simulink model "sampleModel106"  (R2022a)
settings: Solver=VariableStepAuto  StartTime=0.0  StopTime=10.0  RelTol=1e-3
undefined symbols (not defined in the file): DiscIntNeverNeededParam, magnitude, Newton, Raphson
libraries: simulink x379, slpidlib x89
(part 11 of 16)

== system sampleModel106/cfblk80/cfblk10/cfblk8/cfblk12 ==
  cfblk1 : Inport
  cfblk14 : Inport  Port=2
  Action Port : ActionPort  ActionPortLabel=if(u1 >= 0)
  cfblk10 : ComplexToRealImag
  cfblk11 : Constant  Value=[647263997.396458]  SampleTime=1
  cfblk12 : Constant  Value=[-710280411.344243]  SampleTime=1
  cfblk13 : Constant  Value=[-145557332.228966]  SampleTime=1
  cfblk18 : Delay
  cfblk19 : Delay
  cfblk20 : Delay
  cfblk3 : slpidlib/PID Controller (2DOF)  Controller=PID  Form=Parallel  TimeDomain=Discrete-time  UseExternalTs=off  SampleTime=-1  IntegratorMethod=Forward Euler  FilterMethod=Forward Euler  ControllerParametersSource=internal  P=1  I=1  UseKiTs=off  D=0  N=100  UseFilter=on  b=1  c=1  TunerSelectOption=Transfer Function Based (PID Tuner App)  InitialConditionSource=internal  InitialConditionForIntegrator=0  InitialConditionForFilter=0  DifferentiatorICPrevScaledInput=0  ExternalReset=none  TrackingMode=off  Kt=1  LimitOutput=off  SatLimitsSource=internal  UpperSaturationLimit=inf  LowerSaturationLimit=-inf  LinearizeAsGain=off  AntiWindupMode=none  Kb=1  POutMin=[]  POutMax=[]  IOutMin=[]  IOutMax=[]  DOutMin=[]  DOutMax=[]  NOutMin=[]  NOutMax=[]  bOutMin=[]  bOutMax=[]  cOutMin=[]  cOutMax=[]  SumOutMin=[]  SumOutMax=[]  SaturationOutMin=[]  SaturationOutMax=[]  PParamMin=[]  PParamMax=[]  IParamMin=[]  IParamMax=[]  DParamMin=[]  DParamMax=[]  NParamMin=[]  NParamMax=[]  bParamMin=[]  bParamMax=[]  cParamMin=[]  cParamMax=[]  KbParamMin=[]  KbParamMax=[]  KtParamMin=[]  KtParamMax=[]  KbOutMin=[]  KbOutMax=[]  KtOutMin=[]  KtOutMax=[]  IntegratorOutMin=[]  IntegratorOutMax=[]  FilterOutMin=[]  FilterOutMax=[]  SumI1OutMin=[]  SumI1OutMax=[]  SumI2OutMin=[]  SumI2OutMax=[]  SumI3OutMin=[]  SumI3OutMax=[]  SumI4OutMin=[]  SumI4OutMax=[]  SumDOutMin=[]  SumDOutMax=[]  Sum1OutMin=[]  Sum1OutMax=[]  Sum2OutMin=[]  Sum2OutMax=[]  Sum3OutMin=[]  Sum3OutMax=[]  DifferentiatorOutMin=[]  DifferentiatorOutMax=[]  FilterDiffOutCoefMin=[]  FilterDiffOutCoefMax=[]  ReciprocalOutMin=[]  ReciprocalOutMax=[]  SumDenOutMin=[]  SumDenOutMax=[]  SumNumOutMin=[]  SumNumOutMax=[]  DivideOutMin=[]  DivideOutMax=[]  UdiffTsProdOutMin=[]  UdiffTsProdOutMax=[]  NTsProdOutMin=[]  NTsProdOutMax=[]  UintegralTsProdOutMin=[]  UintegralTsProdOutMax=[]  UngainTsProdOutMin=[]  UngainTsProdOutMax=[]  IntegratorContinuousStateAttributes=''  IntegratorStateMustResolveToSignalObject=off  IntegratorRTWStateStorageClass=Auto  FilterContinuousStateAttributes=''  FilterStateMustResolveToSignalObject=off  FilterRTWStateStorageClass=Auto  ParallelPVariant=InternalParameters  IdealPVariant=Disabled  IVariant=InternalParameters  DVariant=InternalParameters  bVariant=InternalParameters  cVariant=InternalParameters  IntegratorVariant=Discrete  SatVariant=Disabled  AWVariant=Passthrough  PCopyVariant=Disabled  TRVariant=Disabled  FdbkBlocksVariant=Forward  IdealPFdbkVariant=Disabled  SatFdbkVariant=Disabled  DerivativeFilterVariant=ForwardEulerFilter  NVariant=InternalParameters  NCopyVariant=Disabled  FilterICVariant=InternalICsFilter  IntegratorICVariant=InternalICs  ExternalResetVariant=Disabled  TRSumVariant=Passthrough  SumFdbkVariant=Disabled  SumVariant=Sum_PID  TsampFilterVariant=InternalTs  TsampNgainVariant=Passthrough  TsampIntegralVariant=Passthrough  ExternalSaturationOutDataTypeStr=Inherit: Same as second input
      settings: SourceProductBaseCode=SL
  cfblk4 : Squeeze
  cfblk5 : Sum  Inputs=+-
  cfblk6 : Sum  Inputs=+-
  cfblk7 : Sum  Inputs=|++
  cfblk8 : Sum  Inputs=+
  cfblk9 : ComplexToRealImag
  cfblk2 : Outport
  cfblk15 : Outport  Port=2
  cfblk16 : Outport  Port=3
  cfblk17 : Outport  Port=4
  wires:
  cfblk9/1 -> cfblk15/1
  cfblk13/1 -> cfblk17/1
  cfblk3/1 -> cfblk5/1
  cfblk14/1 -> cfblk2/1
  cfblk5/1 -> cfblk7/1
  cfblk9/2 -> cfblk10/1, cfblk6/2
  cfblk7/1 -> cfblk8/1
  cfblk8/1 -> cfblk9/1
  cfblk4/1 -> cfblk16/1
  cfblk12/1 -> cfblk7/2
  cfblk11/1 -> cfblk6/1
  cfblk1/1 -> cfblk4/1
  cfblk10/1 -> cfblk18/1
  cfblk18/1 -> cfblk3/1
  cfblk10/2 -> cfblk19/1
  cfblk19/1 -> cfblk3/2
  cfblk6/1 -> cfblk20/1
  cfblk20/1 -> cfblk5/2

== system sampleModel106/cfblk80/cfblk10/cfblk8/cfblk13 ==
  cfblk1 : Inport
  cfblk13 : Inport  Port=2
  cfblk14 : Inport  Port=3
  cfblk15 : Inport  Port=4
  cfblk16 : Inport  Port=5
  cfblk17 : Inport  Port=6
  Action Port : ActionPort  ActionPortLabel=else
  cfblk10 : Constant  Value=[-897843886.378087]  SampleTime=1
  cfblk11 : Constant  Value=[302517880.201654]  SampleTime=1
  cfblk12 : Constant  Value=[630403089.803577]  SampleTime=1
  cfblk3 : simulink/Discrete/Transfer Fcn Real Zero  ZeroZ=0.75  ICPrevInput=0.0  DoSatur=off
      settings: SourceProductBaseCode=SL
  cfblk4 : Reshape
  cfblk5 : Signum
  cfblk6 : Squeeze
  cfblk7 : Bias  Bias=[473175821.464954]  SaturateOnIntegerOverflow=off
  cfblk8 : PermuteDimensions
  cfblk9 : Constant  Value=[-532839668.441266]  SampleTime=1
  cfblk2 : Outport
  wires:
  cfblk11/1 -> cfblk5/1
  cfblk3/1 -> cfblk8/1
  cfblk1/1 -> cfblk3/1
  cfblk9/1 -> cfblk6/1
  cfblk16/1 -> cfblk4/1
  cfblk17/1 -> cfblk2/1
  cfblk15/1 -> cfblk7/1

== system sampleModel106/cfblk80/cfblk10/cfblk8/cfblk6 ==
  cfblk1 : Inport
  cfblk8 : Inport  Port=2
  cfblk9 : Inport  Port=3
  cfblk10 : Inport  Port=4
  cfblk3 : simulink/Discrete/Difference  ICPrevInput=0.0  OutMin=[]  OutMax=[]  OutDataTypeStr=Inherit: Inherit via back propagation  OutDataType=fixdt(1, 16)  OutScaling=2^-10  DoSatur=off
  cfblk4 : Trigonometry
  cfblk5 : Sum  Inputs=+-
  cfblk6 : Constant  Value=[-342792369.326935]  SampleTime=1
  cfblk7 : Constant  Value=[-642019709.076268]  SampleTime=1
  cfblk2 : Outport
  wires:
  cfblk3/1 -> cfblk2/1
  cfblk7/1 -> cfblk5/1
  cfblk10/1 -> cfblk5/2
  cfblk6/1 -> cfblk4/1
  cfblk4/1 -> cfblk3/1

== system sampleModel106/cfblk80/cfblk10/cfblk8/cfblk7 ==
  cfblk1 : Inport
  cfblk15 : Inport  Port=2
  cfblk16 : Inport  Port=3
  cfblk10 : Sum  Inputs=+-
  cfblk11 : Constant  Value=[-15116580.989043]  SampleTime=1
  cfblk12 : Constant  Value=[685298469.116732]  SampleTime=1
  cfblk13 : Constant  Value=[-327896226.329159]  SampleTime=1
  cfblk14 : Constant  Value=[801147045.676296]  SampleTime=1
  cfblk17 : Delay  SampleTime=1
  cfblk3 : Bias  Bias=[-977258308.912659]  SaturateOnIntegerOverflow=off
  cfblk4 : Sum  Inputs=+-
  cfblk5 : Polyval  Coefs=[ +2.081618890e-019, -1.441693666e-014, +4.719686976e-010, -8.536869453e-006, +1.621573104e-001, -8.087801117e+001 ]
  cfblk6 : simulink/Math Operations/MinMax Running Resettable  Function=min  vinit=0.0
  cfblk7 : MinMax  Inputs=2
  cfblk8 : simulink/Math Operations/MinMax Running Resettable  Function=min  vinit=0.0
  cfblk9 : Sin  TimeSource=Use external signal  SampleTime=0
  cfblk2 : Outport
  wires:
  cfblk4/1 -> cfblk7/1
  cfblk13/1 -> cfblk7/2
  cfblk12/1 -> cfblk2/1
  cfblk5/1 -> cfblk4/1
  cfblk3/1 -> cfblk5/1
  cfblk10/1 -> cfblk6/1
  cfblk9/1 -> cfblk6/2
  cfblk14/1 -> cfblk8/1
  cfblk15/1 -> cfblk8/2
  cfblk1/1 -> cfblk3/1
  cfblk8/1 -> cfblk9/1
  cfblk16/1 -> cfblk4/2
  cfblk7/1 -> cfblk10/1
  cfblk6/1 -> cfblk17/1
  cfblk17/1 -> cfblk10/2

== system sampleModel106/cfblk80/cfblk10/cfblk8/cfblk8 ==
  cfblk1 : Inport
  cfblk7 : Inport  Port=2
  cfblk8 : Inport  Port=3
  cfblk9 : Inport  Port=4
  cfblk3 : UnitDelay  HasFrameUpgradeWarning=on
  cfblk4 : Signum
  cfblk5 : Sqrt  Operator=rSqrt  AlgorithmType=Newton-Raphson
  cfblk6 : simulink/Math Operations/MinMax Running Resettable  Function=min  vinit=0.0
  cfblk2 : Outport
  cfblk10 : Outport  Port=2
  cfblk11 : Outport  Port=3
  cfblk12 : Outport  Port=4
  wires:
  cfblk7/1 -> cfblk5/1
  cfblk8/1 -> cfblk3/1
  cfblk3/1 -> cfblk4/1, cfblk2/1
  cfblk6/1 -> cfblk10/1
  cfblk1/1 -> cfblk11/1
  cfblk4/1 -> cfblk12/1
  cfblk5/1 -> cfblk6/1
  cfblk9/1 -> cfblk6/2

== system sampleModel106/cfblk80/cfblk10/cfblk8/cfblk9 ==
  cfblk1 : Inport
  cfblk7 : Inport  Port=2
  cfblk10 : Delay  SampleTime=1
  cfblk11 : Delay  SampleTime=1
  cfblk3 : DiscreteZeroPole  Poles=[0 0.5]  Gain=1
  cfblk4 : UnaryMinus
  cfblk5 : simulink/Math Operations/MinMax Running Resettable  Function=min  vinit=0.0
  cfblk6 : Product  Inputs=**
  cfblk2 : Outport
  cfblk8 : Outport  Port=2
  cfblk9 : Outport  Port=3
  wires:
  cfblk4/1 -> cfblk6/1
  cfblk5/1 -> cfblk2/1, cfblk4/1
  cfblk7/1 -> cfblk8/1
  cfblk6/1 -> cfblk3/1, cfblk11/1
  cfblk1/1 -> cfblk5/1, cfblk9/1
  cfblk3/1 -> cfblk10/1
  cfblk10/1 -> cfblk6/2
  cfblk11/1 -> cfblk5/2

== system sampleModel106/cfblk80/cfblk10/cfblk9/cfblk8 ==
  cfblk1 : Inport
  cfblk7 : Inport  Port=2
  cfblk8 : Inport  Port=3
  cfblk9 : Inport  Port=4
  cfblk3 : simulink/Discrete/Transfer Fcn First Order  PoleZ=0.95  ICPrevOutput=0.0  DoSatur=off
  cfblk4 : Abs  SaturateOnIntegerOverflow=off
  cfblk5 : Sum  Inputs=+
  cfblk6 : Constant  Value=[-161739607.877266]  SampleTime=1
  cfblk2 : Outport
  cfblk10 : Outport  Port=2
  wires:
  cfblk8/1 -> cfblk2/1
  cfblk3/1 -> cfblk5/1
  cfblk4/1 -> cfblk10/1
  cfblk7/1 -> cfblk3/1
  cfblk5/1 -> cfblk4/1

== system sampleModel106/cfblk80/cfblk10/cfblk9/cfblk9 ==
  cfblk1 : Inport
  cfblk3 : simulink/Discrete/Transfer Fcn Lead or Lag  PoleZ=0.95  ZeroZ=0.75  ICPrevOutput=0.0  ICPrevInput=0.0  DoSatur=off
      settings: SourceProductBaseCode=SL
  cfblk4 : Product  Inputs=*
  cfblk5 : Sum
  cfblk6 : Bias  Bias=[-67652395.251411]  SaturateOnIntegerOverflow=off
  cfblk2 : Outport
  cfblk7 : Outport  Port=2
  wires:
  cfblk6/1 -> cfblk5/1
  cfblk1/1 -> cfblk2/1, cfblk3/1, cfblk6/1
  cfblk3/1 -> cfblk4/1
  cfblk5/1 -> cfblk7/1
  cfblk4/1 -> cfblk5/2

== system sampleModel106/cfblk80/cfblk11/cfblk10/cfblk8 ==
  cfblk1 : Inport
  cfblk8 : Inport  Port=2
  cfblk3 : Product  Inputs=**
  cfblk4 : ComplexToRealImag
  cfblk5 : Sqrt  Operator=rSqrt  AlgorithmType=Newton-Raphson
  cfblk6 : ComplexToRealImag
  cfblk7 : Constant  Value=[634238120.262405]  SampleTime=1
  cfblk2 : Outport
  cfblk9 : Outport  Port=2
  wires:
  cfblk7/1 -> cfblk5/1
  cfblk6/1 -> cfblk9/1
  cfblk4/1 -> cfblk3/1
  cfblk1/1 -> cfblk6/1
  cfblk8/1 -> cfblk4/1
  cfblk6/2 -> cfblk2/1
  cfblk5/1 -> cfblk3/2

== system sampleModel106/cfblk80/cfblk11/cfblk10/cfblk9 ==
  cfblk1 : Inport
  cfblk6 : Inport  Port=2
  cfblk3 : Product  Inputs=**
  cfblk4 : Sqrt
  cfblk5 : Constant  Value=[-951789806.354500]  SampleTime=1
  cfblk2 : Outport
  cfblk7 : Outport  Port=2
  wires:
  cfblk4/1 -> cfblk7/1
  cfblk5/1 -> cfblk3/1
  cfblk3/1 -> cfblk4/1
  cfblk6/1 -> cfblk3/2
  cfblk1/1 -> cfblk2/1

== system sampleModel106/cfblk80/cfblk11/cfblk8/cfblk10 ==
  cfblk1 : Inport
  cfblk10 : Inport  Port=2
  cfblk11 : Inport  Port=3
  cfblk13 : Delay  SampleTime=1
  cfblk3 : DiscreteZeroPole  Poles=[0 0.5]  Gain=1
  cfblk4 : Product  Inputs=**
  cfblk5 : Sum  Inputs=+
  cfblk6 : Sqrt
  cfblk7 : simulink/Math Operations/Slider Gain  gain=1  low=0  high=2
  cfblk8 : Gain  Gain=[838906056.735311]
  cfblk9 : Constant  Value=[952501991.848955]  SampleTime=1
  cfblk2 : Outport
  cfblk12 : Outport  Port=2
  wires:
  cfblk9/1 -> cfblk4/1
  cfblk5/1 -> cfblk6/1
  cfblk7/1 -> cfblk3/1
  cfblk8/1 -> cfblk12/1
  cfblk3/1 -> cfblk2/1
  cfblk11/1 -> cfblk7/1
  cfblk4/1 -> cfblk5/1
  cfblk10/1 -> cfblk8/1
  cfblk6/1 -> cfblk13/1
  cfblk13/1 -> cfblk4/2

== system sampleModel106/cfblk80/cfblk11/cfblk8/cfblk11 ==
  cfblk1 : Inport
  cfblk10 : Constant  Value=[-97826944.029732]  SampleTime=1
  cfblk3 : simulink/Math Operations/Slider Gain  gain=1  low=0  high=2
  cfblk4 : Sum  Inputs=|++
  cfblk5 : Sum  Inputs=+-
  cfblk6 : Trigonometry
  cfblk7 : Reshape
  cfblk8 : Constant  Value=[564328220.436240]  SampleTime=1
  cfblk9 : Constant  Value=[-958432842.586397]  SampleTime=1
  cfblk2 : Outport
  cfblk11 : Outport  Port=2
  cfblk12 : Outport  Port=3
  wires:
  cfblk8/1 -> cfblk4/1
  cfblk4/1 -> cfblk7/1
  cfblk10/1 -> cfblk12/1, cfblk3/1
  cfblk6/1 -> cfblk5/1
  cfblk3/1 -> cfblk6/1
  cfblk9/1 -> cfblk5/2
  cfblk1/1 -> cfblk2/1
  cfblk5/1 -> cfblk4/2
  cfblk7/1 -> cfblk11/1

== system sampleModel106/cfblk80/cfblk11/cfblk8/cfblk12 ==
  cfblk1 : Inport
  cfblk10 : Inport  Port=2
  cfblk11 : Inport  Port=3
  cfblk12 : Inport  Port=4
  cfblk14 : Delay  SampleTime=1
  cfblk3 : slpidlib/PID Controller  Controller=PID  Form=Parallel  TimeDomain=Discrete-time  UseExternalTs=off  SampleTime=1  IntegratorMethod=Forward Euler  FilterMethod=Forward Euler  ControllerParametersSource=internal  P=1  I=1  UseKiTs=off  D=0  N=100  UseFilter=on  TunerSelectOption=Transfer Function Based (PID Tuner App)  InitialConditionSource=internal  InitialConditionForIntegrator=0  InitialConditionForFilter=0  DifferentiatorICPrevScaledInput=0  ExternalReset=none  TrackingMode=off  Kt=1  LimitOutput=off  SatLimitsSource=internal  UpperSaturationLimit=inf  LowerSaturationLimit=-inf  LinearizeAsGain=off  AntiWindupMode=none  Kb=1  POutMin=[]  POutMax=[]  IOutMin=[]  IOutMax=[]  DOutMin=[]  DOutMax=[]  NOutMin=[]  NOutMax=[]  SumOutMin=[]  SumOutMax=[]  SaturationOutMin=[]  SaturationOutMax=[]  PParamMin=[]  PParamMax=[]  IParamMin=[]  IParamMax=[]  DParamMin=[]  DParamMax=[]  NParamMin=[]  NParamMax=[]  KbParamMin=[]  KbParamMax=[]  KtParamMin=[]  KtParamMax=[]  KbOutMin=[]  KbOutMax=[]  KtOutMin=[]  KtOutMax=[]  IntegratorOutMin=[]  IntegratorOutMax=[]  FilterOutMin=[]  FilterOutMax=[]  SumI1OutMin=[]  SumI1OutMax=[]  SumI2OutMin=[]  SumI2OutMax=[]  SumI3OutMin=[]  SumI3OutMax=[]  SumI4OutMin=[]  SumI4OutMax=[]  SumDOutMin=[]  SumDOutMax=[]  DifferentiatorOutMin=[]  DifferentiatorOutMax=[]  FilterDiffOutCoefMin=[]  FilterDiffOutCoefMax=[]  ReciprocalOutMin=[]  ReciprocalOutMax=[]  SumDenOutMin=[]  SumDenOutMax=[]  SumNumOutMin=[]  SumNumOutMax=[]  DivideOutMin=[]  DivideOutMax=[]  UdiffTsProdOutMin=[]  UdiffTsProdOutMax=[]  NTsProdOutMin=[]  NTsProdOutMax=[]  UintegralTsProdOutMin=[]  UintegralTsProdOutMax=[]  UngainTsProdOutMin=[]  UngainTsProdOutMax=[]  IntegratorContinuousStateAttributes=''  IntegratorStateMustResolveToSignalObject=off  IntegratorRTWStateStorageClass=Auto  FilterContinuousStateAttributes=''  FilterStateMustResolveToSignalObject=off  FilterRTWStateStorageClass=Auto  ParallelPVariant=InternalParameters  IdealPVariant=Disabled  IVariant=InternalParameters  DVariant=InternalParameters  IntegratorVariant=Discrete  SatVariant=Disabled  AWVariant=Passthrough  PCopyVariant=Disabled  TRVariant=Disabled  FdbkBlocksVariant=Forward  IdealPFdbkVariant=Disabled  SatFdbkVariant=Disabled  DerivativeFilterVariant=ForwardEulerFilter  NVariant=InternalParameters  NCopyVariant=Disabled  FilterICVariant=InternalICsFilter  IntegratorICVariant=InternalICs  ExternalResetVariant=Disabled  TRSumVariant=Passthrough  SumFdbkVariant=Disabled  SumVariant=Sum_PID  TsampFilterVariant=InternalTs  TsampNgainVariant=Passthrough  TsampIntegralVariant=Passthrough  ExternalSaturationOutDataTypeStr=Inherit: Same as second input  aMode=0
  cfblk4 : Math  Operator=magnitude^2
  cfblk5 : Squeeze
  cfblk6 : Sum  Inputs=-+
  cfblk7 : simulink/Math Operations/Slider Gain  gain=1  low=0  high=2
  cfblk8 : PermuteDimensions
  cfblk9 : Constant  Value=[355141637.645424]  SampleTime=1
  cfblk2 : Outport
  cfblk13 : Outport  Port=2
  wires:
  cfblk11/1 -> cfblk4/1
  cfblk10/1 -> cfblk2/1
  cfblk12/1 -> cfblk8/1
  cfblk3/1 -> cfblk6/1
  cfblk1/1 -> cfblk13/1
  cfblk8/1 -> cfblk7/1
  cfblk4/1 -> cfblk6/2
  cfblk6/1 -> cfblk5/1
  cfblk5/1 -> cfblk14/1
  cfblk14/1 -> cfblk3/1

== system sampleModel106/cfblk80/cfblk11/cfblk8/cfblk7 ==
  cfblk1 : Inport
  cfblk7 : Inport  Port=2
  cfblk3 : simulink/Discrete/Difference  ICPrevInput=0.0  OutMin=[]  OutMax=[]  OutDataTypeStr=Inherit: Inherit via back propagation  OutDataType=fixdt(1, 16)  OutScaling=2^-10  DoSatur=off
  cfblk4 : Constant  Value=[-388420622.706026]  SampleTime=1
  cfblk5 : Constant  Value=[174605432.981955]  SampleTime=1
  cfblk6 : Constant  Value=[-811978133.934877]  SampleTime=1
  cfblk2 : Outport
  wires:
  cfblk1/1 -> cfblk2/1
  cfblk6/1 -> cfblk3/1

== system sampleModel106/cfblk80/cfblk11/cfblk8/cfblk8 ==
  cfblk1 : Inport
  cfblk13 : Inport  Port=2
  cfblk14 : Inport  Port=3
  cfblk15 : Inport  Port=4
  cfblk10 : Product
  cfblk11 : Signum
  cfblk12 : Polyval  Coefs=[ +2.081618890e-019, -1.441693666e-014, +4.719686976e-010, -8.536869453e-006, +1.621573104e-001, -8.087801117e+001 ]
  cfblk16 : Delay  SampleTime=1
  cfblk3 : simulink/Discrete/Tapped Delay  vinit=0.0  samptime=-1  NumDelays=1  DelayOrder=Oldest  includeCurrent=off
  cfblk4 : simulink/Discrete/Transfer Fcn Lead or Lag  PoleZ=0.95  ZeroZ=0.75  ICPrevOutput=0.0  ICPrevInput=0.0  DoSatur=off
      settings: SourceProductBaseCode=SL
  cfblk5 : slpidlib/PID Controller (2DOF)  Controller=PID  Form=Parallel  TimeDomain=Discrete-time  UseExternalTs=off  SampleTime=1  IntegratorMethod=Forward Euler  FilterMethod=Forward Euler  ControllerParametersSource=internal  P=1  I=1  UseKiTs=off  D=0  N=100  UseFilter=on  b=1  c=1  TunerSelectOption=Transfer Function Based (PID Tuner App)  InitialConditionSource=internal  InitialConditionForIntegrator=0  InitialConditionForFilter=0  DifferentiatorICPrevScaledInput=0  ExternalReset=none  TrackingMode=off  Kt=1  LimitOutput=off  SatLimitsSource=internal  UpperSaturationLimit=inf  LowerSaturationLimit=-inf  LinearizeAsGain=off  AntiWindupMode=none  Kb=1  POutMin=[]  POutMax=[]  IOutMin=[]  IOutMax=[]  DOutMin=[]  DOutMax=[]  NOutMin=[]  NOutMax=[]  bOutMin=[]  bOutMax=[]  cOutMin=[]  cOutMax=[]  SumOutMin=[]  SumOutMax=[]  SaturationOutMin=[]  SaturationOutMax=[]  PParamMin=[]  PParamMax=[]  IParamMin=[]  IParamMax=[]  DParamMin=[]  DParamMax=[]  NParamMin=[]  NParamMax=[]  bParamMin=[]  bParamMax=[]  cParamMin=[]  cParamMax=[]  KbParamMin=[]  KbParamMax=[]  KtParamMin=[]  KtParamMax=[]  KbOutMin=[]  KbOutMax=[]  KtOutMin=[]  KtOutMax=[]  IntegratorOutMin=[]  IntegratorOutMax=[]  FilterOutMin=[]  FilterOutMax=[]  SumI1OutMin=[]  SumI1OutMax=[]  SumI2OutMin=[]  SumI2OutMax=[]  SumI3OutMin=[]  SumI3OutMax=[]  SumI4OutMin=[]  SumI4OutMax=[]  SumDOutMin=[]  SumDOutMax=[]  Sum1OutMin=[]  Sum1OutMax=[]  Sum2OutMin=[]  Sum2OutMax=[]  Sum3OutMin=[]  Sum3OutMax=[]  DifferentiatorOutMin=[]  DifferentiatorOutMax=[]  FilterDiffOutCoefMin=[]  FilterDiffOutCoefMax=[]  ReciprocalOutMin=[]  ReciprocalOutMax=[]  SumDenOutMin=[]  SumDenOutMax=[]  SumNumOutMin=[]  SumNumOutMax=[]  DivideOutMin=[]  DivideOutMax=[]  UdiffTsProdOutMin=[]  UdiffTsProdOutMax=[]  NTsProdOutMin=[]  NTsProdOutMax=[]  UintegralTsProdOutMin=[]  UintegralTsProdOutMax=[]  UngainTsProdOutMin=[]  UngainTsProdOutMax=[]  IntegratorContinuousStateAttributes=''  IntegratorStateMustResolveToSignalObject=off  IntegratorRTWStateStorageClass=Auto  FilterContinuousStateAttributes=''  FilterStateMustResolveToSignalObject=off  FilterRTWStateStorageClass=Auto  ParallelPVariant=InternalParameters  IdealPVariant=Disabled  IVariant=InternalParameters  DVariant=InternalParameters  bVariant=InternalParameters  cVariant=InternalParameters  IntegratorVariant=Discrete  SatVariant=Disabled  AWVariant=Passthrough  PCopyVariant=Disabled  TRVariant=Disabled  FdbkBlocksVariant=Forward  IdealPFdbkVariant=Disabled  SatFdbkVariant=Disabled  DerivativeFilterVariant=ForwardEulerFilter  NVariant=InternalParameters  NCopyVariant=Disabled  FilterICVariant=InternalICsFilter  IntegratorICVariant=InternalICs  ExternalResetVariant=Disabled  TRSumVariant=Passthrough  SumFdbkVariant=Disabled  SumVariant=Sum_PID  TsampFilterVariant=InternalTs  TsampNgainVariant=Passthrough  TsampIntegralVariant=Passthrough  ExternalSaturationOutDataTypeStr=Inherit: Same as second input
      settings: SourceProductBaseCode=SL
  cfblk6 : Delay  DelayLengthSource=Input port  SampleTime=1
      settings: InputPortMap=u0,p1
  cfblk7 : simulink/Discrete/Transfer Fcn Real Zero  ZeroZ=0.75  ICPrevInput=0.0  DoSatur=off
      settings: SourceProductBaseCode=SL
  cfblk8 : ComplexToMagnitudeAngle
  cfblk9 : ComplexToMagnitudeAngle
  cfblk2 : Outport
  wires:
  cfblk5/1 -> cfblk12/1
  cfblk6/1 -> cfblk2/1
  cfblk12/1 -> cfblk9/1
  cfblk4/1 -> cfblk3/1
  cfblk8/1 -> cfblk10/2
  cfblk11/1 -> cfblk8/1
  cfblk13/1 -> cfblk4/1
  cfblk1/1 -> cfblk11/1
  cfblk7/1 -> cfblk5/1
  cfblk10/1 -> cfblk5/2
  cfblk15/1 -> cfblk7/1
  cfblk3/1 -> cfblk6/1
  cfblk8/2 -> cfblk6/2
  cfblk9/1 -> cfblk16/1
  cfblk16/1 -> cfblk10/1

== system sampleModel106/cfblk80/cfblk11/cfblk8/cfblk9 ==
  cfblk1 : Inport
  cfblk11 : Inport  Port=2
  cfblk12 : Inport  Port=3
  cfblk13 : Inport  Port=4
  cfblk14 : Inport  Port=5
  cfblk10 : Math  Operator=rem
  cfblk3 : UnitDelay  HasFrameUpgradeWarning=on
  cfblk4 : Sqrt  Operator=rSqrt  AlgorithmType=Newton-Raphson
  cfblk5 : Assignment  DiagnosticForDimensions=Warning  IndexOptions=Index vector (dialog)  Indices=1  OutputSizes=1
  cfblk6 : Sqrt
  cfblk7 : UnaryMinus
  cfblk8 : UnaryMinus
  cfblk9 : simulink/Math Operations/Slider Gain  gain=1  low=0  high=2
  cfblk2 : Outport
  cfblk15 : Outport  Port=2
  wires:
  cfblk4/1 -> cfblk3/1
  cfblk8/1 -> cfblk4/1
  cfblk14/1 -> cfblk9/1
  cfblk12/1 -> cfblk8/1
  cfblk6/1 -> cfblk5/1
  cfblk13/1 -> cfblk6/1
  cfblk3/1 -> cfblk10/1
  cfblk1/1 -> cfblk10/2
  cfblk10/1 -> cfblk7/1
  cfblk9/1 -> cfblk15/1
  cfblk7/1 -> cfblk5/2
  cfblk5/1 -> cfblk2/1

== system sampleModel106/cfblk80/cfblk11/cfblk9/cfblk10 ==
  cfblk1 : Inport
  cfblk11 : Inport  Port=2
  cfblk12 : Inport  Port=3
  cfblk13 : Inport  Port=4
  cfblk14 : Inport  Port=5
  cfblk15 : Inport  Port=6
  cfblk16 : Inport  Port=7
  cfblk17 : Inport  Port=8
  cfblk10 : Constant  Value=[597382061.166355]  SampleTime=1
  cfblk3 : simulink/Discrete/Difference  ICPrevInput=0.0  OutMin=[]  OutMax=[]  OutDataTypeStr=Inherit: Inherit via back propagation  OutDataType=fixdt(1, 16)  OutScaling=2^-10  DoSatur=off
  cfblk4 : DiscreteIntegrator  ICPrevOutput=DiscIntNeverNeededParam  ICPrevScaledInput=DiscIntNeverNeededParam
  cfblk5 : simulink/Math Operations/MinMax Running Resettable  Function=min  vinit=0.0
  cfblk6 : Sin  TimeSource=Use external signal  SampleTime=0
  cfblk7 : Rounding
  cfblk8 : Sum  Inputs=-+
  cfblk9 : UnaryMinus
  cfblk2 : Outport
  wires:
  cfblk12/1 -> cfblk9/1
  cfblk10/1 -> cfblk8/1
  cfblk13/1 -> cfblk3/1
  cfblk11/1 -> cfblk7/1
  cfblk9/1 -> cfblk5/1
  cfblk4/1 -> cfblk8/2
  cfblk6/1 -> cfblk2/1
  cfblk17/1 -> cfblk6/1
  cfblk1/1 -> cfblk4/1
  cfblk14/1 -> cfblk5/2

== system sampleModel106/cfblk80/cfblk11/cfblk9/cfblk11 ==
  cfblk1 : Inport
  cfblk13 : Inport  Port=2
  cfblk14 : Inport  Port=3
  cfblk10 : Sum  Inputs=+
  cfblk11 : ComplexToRealImag
  cfblk12 : simulink/Math Operations/MinMax Running Resettable  Function=min  vinit=0.0
  cfblk15 : Delay  SampleTime=1
  cfblk16 : Delay  SampleTime=1
  cfblk3 : simulink/Discrete/Tapped Delay  vinit=0.0  samptime=-1  NumDelays=1  DelayOrder=Oldest  includeCurrent=off
  cfblk4 : DotProduct  OutDataTypeStr=Inherit: Inherit via internal rule
  cfblk5 : Gain  Gain=[-848370394.486433]
  cfblk6 : Sqrt
  cfblk7 : MinMax  Function=max  Inputs=2
  cfblk8 : Sum  Inputs=+
  cfblk9 : UnaryMinus
  cfblk2 : Outport
  wires:
  cfblk8/1 -> cfblk5/1
  cfblk1/1 -> cfblk11/1
  cfblk3/1 -> cfblk9/1
  cfblk5/1 -> cfblk4/1
  cfblk13/1 -> cfblk8/1
  cfblk4/1 -> cfblk7/1
  cfblk6/1 -> cfblk2/1
  cfblk14/1 -> cfblk12/1
  cfblk11/1 -> cfblk10/1
  cfblk11/2 -> cfblk6/1
  cfblk10/1 -> cfblk4/2
  cfblk7/1 -> cfblk12/2
  cfblk12/1 -> cfblk15/1
  cfblk15/1 -> cfblk7/2
  cfblk9/1 -> cfblk16/1
  cfblk16/1 -> cfblk3/1

== system sampleModel106/cfblk80/cfblk11/cfblk9/cfblk12 ==
  cfblk1 : Inport
  cfblk10 : Inport  Port=2
  cfblk11 : Inport  Port=3
  cfblk12 : Inport  Port=4
  cfblk13 : Inport  Port=5
  cfblk3 : Bias  Bias=[483311717.841086]  SaturateOnIntegerOverflow=off
  cfblk4 : Product  Inputs=**
  cfblk5 : simulink/Math Operations/MinMax Running Resettable  Function=min  vinit=0.0
  cfblk6 : ComplexToRealImag
  cfblk7 : Constant  Value=[-122869408.637537]  SampleTime=1
  cfblk8 : Constant  Value=[744089933.160599]  SampleTime=1
  cfblk9 : Constant  Value=[488267635.496395]  SampleTime=1
  cfblk2 : Outport
  cfblk14 : Outport  Port=2
  cfblk15 : Outport  Port=3
  wires:
  cfblk13/1 -> cfblk5/1
  cfblk6/1 -> cfblk2/1
  cfblk6/2 -> cfblk4/1
  cfblk8/1 -> cfblk14/1
  cfblk9/1 -> cfblk15/1
  cfblk11/1 -> cfblk4/2
  cfblk1/1 -> cfblk6/1
  cfblk3/1 -> cfblk5/2
  cfblk10/1 -> cfblk3/1

== system sampleModel106/cfblk80/cfblk11/cfblk9/cfblk13 ==
  cfblk1 : Inport
  cfblk12 : Inport  Port=2
  cfblk13 : Inport  Port=3
  cfblk14 : Inport  Port=4
  cfblk15 : Inport  Port=5
  cfblk10 : Constant  Value=[-835516922.438338]  SampleTime=1
  cfblk11 : Constant  Value=[-312297949.781857]  SampleTime=1
  cfblk3 : DiscreteFilter  SampleTime=1
  cfblk4 : simulink/Discrete/Transfer Fcn First Order  PoleZ=0.95  ICPrevOutput=0.0  DoSatur=off
  cfblk5 : Delay  ShowEnablePort=on  SampleTime=1
      settings: InputPortMap=u0,e6
  cfblk6 : ComplexToMagnitudeAngle
  cfblk7 : UnaryMinus
  cfblk8 : Gain  Gain=[-280348238.602837]
  cfblk9 : ComplexToMagnitudeAngle
  cfblk2 : Outport
  cfblk16 : Outport  Port=2
  wires:
  cfblk3/1 -> cfblk6/1
  cfblk6/1 -> cfblk8/1
  cfblk12/1 -> cfblk7/1
  cfblk11/1 -> cfblk4/1
  cfblk5/1 -> cfblk2/1
  cfblk9/1 -> cfblk5/1
  cfblk14/1 -> cfblk9/1
  cfblk9/2 -> cfblk16/1
  cfblk7/1 -> cfblk3/1
  cfblk13/1 -> cfblk5/2

== system sampleModel106/cfblk80/cfblk11/cfblk9/cfblk8 ==
  cfblk1 : Inport
  cfblk11 : Inport  Port=2
  cfblk12 : Inport  Port=3
  cfblk10 : Constant  Value=[117047349.027071]  SampleTime=1
  cfblk3 : Math
  cfblk4 : simulink/Math Operations/Slider Gain  gain=1  low=0  high=2
  cfblk5 : Sin  TimeSource=Use external signal  SampleTime=0
  cfblk6 : Signum
  cfblk7 : Sum  Inputs=+
  cfblk8 : Reshape
  cfblk9 : Constant  Value=[760432113.046271]  SampleTime=1
  cfblk2 : Outport
  cfblk13 : Outport  Port=2
  wires:
  cfblk8/1 -> cfblk5/1
  cfblk12/1 -> cfblk2/1
  cfblk9/1 -> cfblk6/1
  cfblk4/1 -> cfblk13/1
  cfblk10/1 -> cfblk3/1
  cfblk11/1 -> cfblk8/1
  cfblk6/1 -> cfblk7/1
  cfblk7/1 -> cfblk4/1

== system sampleModel106/cfblk80/cfblk11/cfblk9/cfblk9 ==
  cfblk1 : Inport
  cfblk11 : Inport  Port=2
  cfblk10 : Constant  Value=[-210483697.509697]  SampleTime=1
  cfblk3 : DiscreteFilter  SampleTime=1
  cfblk4 : Delay  ShowEnablePort=on  SampleTime=1
      settings: InputPortMap=u0,e6
  cfblk5 : ComplexToMagnitudeAngle
  cfblk6 : Sum  Inputs=+-
  cfblk7 : DotProduct  OutDataTypeStr=Inherit: Inherit via internal rule
  cfblk8 : Constant  Value=[784975148.255530]  SampleTime=1
  cfblk9 : Constant  Value=[922008324.366607]  SampleTime=1
  cfblk2 : Outport
  cfblk12 : Outport  Port=2
  wires:
  cfblk7/1 -> cfblk2/1
  cfblk1/1 -> cfblk5/1
  cfblk3/1 -> cfblk4/1
  cfblk5/1 -> cfblk4/2
  cfblk6/1 -> cfblk3/1
  cfblk8/1 -> cfblk6/1
  cfblk11/1 -> cfblk12/1
  cfblk10/1 -> cfblk6/2
  cfblk5/2 -> cfblk7/1
  cfblk9/1 -> cfblk7/2

== system sampleModel106/cfblk80/cfblk12/cfblk9/cfblk6 ==
  cfblk1 : Inport
  cfblk3 : Sqrt  Operator=rSqrt  AlgorithmType=Newton-Raphson
  cfblk4 : Sqrt
  cfblk5 : Squeeze
  cfblk6 : Sqrt  Operator=rSqrt  AlgorithmType=Newton-Raphson
  cfblk7 : Constant  Value=[374698804.406343]  SampleTime=1
  cfblk8 : Delay  SampleTime=1
  cfblk2 : Outport
  wires:
  cfblk4/1 -> cfblk5/1
  cfblk1/1 -> cfblk6/1
  cfblk3/1 -> cfblk2/1
  cfblk7/1 -> cfblk3/1
  cfblk5/1 -> cfblk8/1
  cfblk8/1 -> cfblk4/1

== system sampleModel106/cfblk80/cfblk12/cfblk9/cfblk8 ==
  cfblk1 : Inport
  cfblk12 : Inport  Port=2
  Action Port : ActionPort  ActionPortLabel=if(u1 >= 0)
  cfblk10 : Constant  Value=[284006111.438589]  SampleTime=1
  cfblk11 : Constant  Value=[927823059.958068]  SampleTime=1
  cfblk3 : Abs  SaturateOnIntegerOverflow=off
  cfblk4 : Sqrt  Operator=rSqrt  AlgorithmType=Newton-Raphson
  cfblk5 : MinMax  Inputs=2
  cfblk6 : Sum
  cfblk7 : simulink/Math Operations/Slider Gain  gain=1  low=0  high=2
  cfblk8 : Constant  Value=[168525030.043507]  SampleTime=1
  cfblk9 : Constant  Value=[754726346.565760]  SampleTime=1
  cfblk2 : Outport
  cfblk13 : Outport  Port=2
  cfblk14 : Outport  Port=3
  wires:
  cfblk7/1 -> cfblk13/1
  cfblk5/1 -> cfblk7/1
  cfblk9/1 -> cfblk4/1
  cfblk3/1 -> cfblk14/1
  cfblk11/1 -> cfblk6/1
  cfblk4/1 -> cfblk5/1
  cfblk6/1 -> cfblk5/2
  cfblk8/1 -> cfblk3/1
  cfblk1/1 -> cfblk6/2
  cfblk10/1 -> cfblk2/1

== system sampleModel106/cfblk80/cfblk12/cfblk9/cfblk9 ==
  cfblk1 : Inport
  cfblk9 : Inport  Port=2
  cfblk10 : Inport  Port=3
  cfblk11 : Inport  Port=4
  cfblk12 : Inport  Port=5
  cfblk13 : Inport  Port=6
  Action Port : ActionPort  ActionPortLabel=else
  cfblk3 : simulink/Discrete/Difference  ICPrevInput=0.0  OutMin=[]  OutMax=[]  OutDataTypeStr=Inherit: Inherit via back propagation  OutDataType=fixdt(1, 16)  OutScaling=2^-10  DoSatur=off
  cfblk4 : simulink/Discrete/Difference  ICPrevInput=0.0  OutMin=[]  OutMax=[]  OutDataTypeStr=Inherit: Inherit via back propagation  OutDataType=fixdt(1, 16)  OutScaling=2^-10  DoSatur=off
  cfblk5 : PermuteDimensions
  cfblk6 : Gain  Gain=[723531019.023412]
  cfblk7 : Abs  SaturateOnIntegerOverflow=off
  cfblk8 : ComplexToRealImag
  cfblk2 : Outport
  cfblk14 : Outport  Port=2
  cfblk15 : Outport  Port=3
  cfblk16 : Outport  Port=4
  wires:
  cfblk10/1 -> cfblk8/1
  cfblk4/1 -> cfblk3/1
  cfblk12/1 -> cfblk14/1
  cfblk3/1 -> cfblk6/1
  cfblk8/1 -> cfblk2/1
  cfblk8/2 -> cfblk5/1
  cfblk11/1 -> cfblk16/1
  cfblk13/1 -> cfblk7/1
  cfblk1/1 -> cfblk15/1
  cfblk9/1 -> cfblk4/1

== system sampleModel106/cfblk80/cfblk8/cfblk7/cfblk6 ==
  cfblk1 : Inport
  cfblk9 : Inport  Port=2
  cfblk10 : Inport  Port=3
  cfblk11 : Inport  Port=4
  cfblk3 : Squeeze
  cfblk4 : ComplexToRealImag
  cfblk5 : Trigonometry
  cfblk6 : Constant  Value=[-942400989.211729]  SampleTime=1
  cfblk7 : Constant  Value=[976415821.440071]  SampleTime=1
  cfblk8 : Constant  Value=[-323435047.681891]  SampleTime=1
  cfblk2 : Outport
  cfblk12 : Outport  Port=2
  wires:
  cfblk7/1 -> cfblk3/1
  cfblk6/1 -> cfblk12/1
  cfblk8/1 -> cfblk2/1
  cfblk3/1 -> cfblk5/1
  cfblk9/1 -> cfblk4/1

== system sampleModel106/cfblk80/cfblk8/cfblk8/cfblk6 ==
  cfblk1 : Inport
  cfblk11 : Inport  Port=2
  cfblk12 : Inport  Port=3
  cfblk13 : Inport  Port=4
  cfblk14 : Inport  Port=5
  cfblk10 : Constant  Value=[-729602414.884745]  SampleTime=1
  cfblk3 : Delay  SampleTime=1
  cfblk4 : DotProduct  OutDataTypeStr=Inherit: Inherit via internal rule
  cfblk5 : Polyval  Coefs=[ +2.081618890e-019, -1.441693666e-014, +4.719686976e-010, -8.536869453e-006, +1.621573104e-001, -8.087801117e+001 ]
  cfblk6 : UnaryMinus
  cfblk7 : Constant  Value=[511434019.855518]  SampleTime=1
  cfblk8 : Constant  Value=[87979230.504950]  SampleTime=1
  cfblk9 : Constant  Value=[115232985.531480]  SampleTime=1
  cfblk2 : Outport
  wires:
  cfblk8/1 -> cfblk4/1
  cfblk13/1 -> cfblk2/1
  cfblk9/1 -> cfblk4/2
  cfblk1/1 -> cfblk5/1
  cfblk14/1 -> cfblk3/1
  cfblk12/1 -> cfblk6/1

== system sampleModel106/cfblk80/cfblk8/cfblk8/cfblk7 ==
  cfblk1 : Inport
  cfblk10 : Inport  Port=2
  cfblk11 : Inport  Port=3
  cfblk12 : Inport  Port=4
  cfblk13 : Inport  Port=5
  cfblk3 : DiscreteZeroPole  Poles=[0 0.5]  Gain=1
  cfblk4 : Signum
  cfblk5 : simulink/Math Operations/MinMax Running Resettable  Function=min  vinit=0.0
  cfblk6 : Sum  Inputs=+
  cfblk7 : Sqrt
  cfblk8 : Constant  Value=[-737395737.383203]  SampleTime=1
  cfblk9 : Constant  Value=[407941909.665505]  SampleTime=1
  cfblk2 : Outport
  cfblk14 : Outport  Port=2
  wires:
  cfblk5/1 -> cfblk3/1
  cfblk11/1 -> cfblk6/1
  cfblk10/1 -> cfblk4/1
  cfblk9/1 -> cfblk7/1
  cfblk8/1 -> cfblk2/1
  cfblk1/1 -> cfblk5/1
  cfblk6/1 -> cfblk14/1
  cfblk4/1 -> cfblk5/2

== system sampleModel106/cfblk80/cfblk9/cfblk11/cfblk9 ==
  cfblk1 : Inport
  cfblk12 : Inport  Port=2
  cfblk13 : Inport  Port=3
  cfblk10 : Signum
  cfblk11 : Constant  Value=[-878725308.110916]  SampleTime=1
  cfblk17 : Delay
  cfblk18 : Delay
  cfblk3 : simulink/Discrete/Difference  ICPrevInput=0.0  OutMin=[]  OutMax=[]  OutDataTypeStr=Inherit: Inherit via back propagation  OutDataType=fixdt(1, 16)  OutScaling=2^-10  DoSatur=off
  cfblk4 : DiscreteTransferFcn
  cfblk5 : simulink/Discrete/Transfer Fcn First Order  PoleZ=0.95  ICPrevOutput=0.0  DoSatur=off
  cfblk6 : slpidlib/PID Controller (2DOF)  Controller=PID  Form=Parallel  TimeDomain=Discrete-time  UseExternalTs=off  SampleTime=-1  IntegratorMethod=Forward Euler  FilterMethod=Forward Euler  ControllerParametersSource=internal  P=1  I=1  UseKiTs=off  D=0  N=100  UseFilter=on  b=1  c=1  TunerSelectOption=Transfer Function Based (PID Tuner App)  InitialConditionSource=internal  InitialConditionForIntegrator=0  InitialConditionForFilter=0  DifferentiatorICPrevScaledInput=0  ExternalReset=none  TrackingMode=off  Kt=1  LimitOutput=off  SatLimitsSource=internal  UpperSaturationLimit=inf  LowerSaturationLimit=-inf  LinearizeAsGain=off  AntiWindupMode=none  Kb=1  POutMin=[]  POutMax=[]  IOutMin=[]  IOutMax=[]  DOutMin=[]  DOutMax=[]  NOutMin=[]  NOutMax=[]  bOutMin=[]  bOutMax=[]  cOutMin=[]  cOutMax=[]  SumOutMin=[]  SumOutMax=[]  SaturationOutMin=[]  SaturationOutMax=[]  PParamMin=[]  PParamMax=[]  IParamMin=[]  IParamMax=[]  DParamMin=[]  DParamMax=[]  NParamMin=[]  NParamMax=[]  bParamMin=[]  bParamMax=[]  cParamMin=[]  cParamMax=[]  KbParamMin=[]  KbParamMax=[]  KtParamMin=[]  KtParamMax=[]  KbOutMin=[]  KbOutMax=[]  KtOutMin=[]  KtOutMax=[]  IntegratorOutMin=[]  IntegratorOutMax=[]  FilterOutMin=[]  FilterOutMax=[]  SumI1OutMin=[]  SumI1OutMax=[]  SumI2OutMin=[]  SumI2OutMax=[]  SumI3OutMin=[]  SumI3OutMax=[]  SumI4OutMin=[]  SumI4OutMax=[]  SumDOutMin=[]  SumDOutMax=[]  Sum1OutMin=[]  Sum1OutMax=[]  Sum2OutMin=[]  Sum2OutMax=[]  Sum3OutMin=[]  Sum3OutMax=[]  DifferentiatorOutMin=[]  DifferentiatorOutMax=[]  FilterDiffOutCoefMin=[]  FilterDiffOutCoefMax=[]  ReciprocalOutMin=[]  ReciprocalOutMax=[]  SumDenOutMin=[]  SumDenOutMax=[]  SumNumOutMin=[]  SumNumOutMax=[]  DivideOutMin=[]  DivideOutMax=[]  UdiffTsProdOutMin=[]  UdiffTsProdOutMax=[]  NTsProdOutMin=[]  NTsProdOutMax=[]  UintegralTsProdOutMin=[]  UintegralTsProdOutMax=[]  UngainTsProdOutMin=[]  UngainTsProdOutMax=[]  IntegratorContinuousStateAttributes=''  IntegratorStateMustResolveToSignalObject=off  IntegratorRTWStateStorageClass=Auto  FilterContinuousStateAttributes=''  FilterStateMustResolveToSignalObject=off  FilterRTWStateStorageClass=Auto  ParallelPVariant=InternalParameters  IdealPVariant=Disabled  IVariant=InternalParameters  DVariant=InternalParameters  bVariant=InternalParameters  cVariant=InternalParameters  IntegratorVariant=Discrete  SatVariant=Disabled  AWVariant=Passthrough  PCopyVariant=Disabled  TRVariant=Disabled  FdbkBlocksVariant=Forward  IdealPFdbkVariant=Disabled  SatFdbkVariant=Disabled  DerivativeFilterVariant=ForwardEulerFilter  NVariant=InternalParameters  NCopyVariant=Disabled  FilterICVariant=InternalICsFilter  IntegratorICVariant=InternalICs  ExternalResetVariant=Disabled  TRSumVariant=Passthrough  SumFdbkVariant=Disabled  SumVariant=Sum_PID  TsampFilterVariant=InternalTs  TsampNgainVariant=Passthrough  TsampIntegralVariant=Passthrough  ExternalSaturationOutDataTypeStr=Inherit: Same as second input
      settings: SourceProductBaseCode=SL
  cfblk7 : DiscreteStateSpace  SampleTime=-1
  cfblk8 : PermuteDimensions
  cfblk9 : Abs  SaturateOnIntegerOverflow=off
  cfblk2 : Outport
  cfblk14 : Outport  Port=2
  cfblk15 : Outport  Port=3
  cfblk16 : Outport  Port=4
  wires:
  cfblk4/1 -> cfblk7/1
  cfblk9/1 -> cfblk6/1
  cfblk10/1 -> cfblk14/1
  cfblk6/1 -> cfblk16/1
  cfblk13/1 -> cfblk3/1
  cfblk12/1 -> cfblk6/2
  cfblk5/1 -> cfblk8/1
  cfblk3/1 -> cfblk9/1
  cfblk1/1 -> cfblk15/1, cfblk10/1
  cfblk11/1 -> cfblk2/1
  cfblk7/1 -> cfblk17/1
  cfblk17/1 -> cfblk4/1
  cfblk8/1 -> cfblk18/1
  cfblk18/1 -> cfblk5/1

== system sampleModel106/cfblk80/cfblk9/cfblk12/cfblk10 ==
  cfblk1 : Inport
  cfblk9 : Inport  Port=2
  cfblk10 : Inport  Port=3
  cfblk11 : Inport  Port=4
  cfblk14 : Delay
  cfblk15 : Delay
  cfblk3 : Delay  ShowEnablePort=on
      settings: InputPortMap=u0,e6
  cfblk4 : ComplexToMagnitudeAngle
  cfblk5 : Sqrt  Operator=rSqrt  AlgorithmType=Newton-Raphson
  cfblk6 : DotProduct  OutDataTypeStr=Inherit: Inherit via internal rule
  cfblk7 : Rounding
  cfblk8 : Gain  Gain=[-554037054.159889]
  cfblk2 : Outport
  cfblk12 : Outport  Port=2
  cfblk13 : Outport  Port=3
  wires:
  cfblk11/1 -> cfblk13/1
  cfblk1/1 -> cfblk3/1
  cfblk9/1 -> cfblk3/2
  cfblk3/1 -> cfblk2/1
  cfblk10/1 -> cfblk8/1
  cfblk4/1 -> cfblk12/1
  cfblk4/2 -> cfblk5/1
  cfblk8/1 -> cfblk6/2
  cfblk6/1 -> cfblk7/1
  cfblk5/1 -> cfblk14/1
  cfblk14/1 -> cfblk4/1
  cfblk7/1 -> cfblk15/1
  cfblk15/1 -> cfblk6/1

== system sampleModel106/cfblk80/cfblk9/cfblk12/cfblk11 ==
  cfblk1 : Inport
  cfblk8 : Inport  Port=2
  cfblk9 : Inport  Port=3
  cfblk10 : Inport  Port=4
  cfblk3 : Sum  Inputs=|++
  cfblk4 : simulink/Math Operations/Slider Gain  gain=1  low=0  high=2
  cfblk5 : ComplexToMagnitudeAngle
  cfblk6 : Constant  Value=[791724712.152659]  SampleTime=1
  cfblk7 : Constant  Value=[-886024125.216931]  SampleTime=1
  cfblk2 : Outport
  cfblk11 : Outport  Port=2
  wires:
  cfblk10/1 -> cfblk3/1
  cfblk8/1 -> cfblk5/1
  cfblk9/1 -> cfblk11/1
  cfblk7/1 -> cfblk4/1
  cfblk5/1 -> cfblk2/1
  cfblk5/2 -> cfblk3/2

== system sampleModel106/cfblk80/cfblk9/cfblk12/cfblk6 ==
  cfblk1 : Inport
  cfblk3 : DiscreteZeroPole  Poles=[0 0.5]  Gain=1  SampleTime=-1
  cfblk4 : ComplexToRealImag
  cfblk5 : Polyval  Coefs=[ +2.081618890e-019, -1.441693666e-014, +4.719686976e-010, -8.536869453e-006, +1.621573104e-001, -8.087801117e+001 ]
  cfblk6 : Reshape
  cfblk7 : Rounding
  cfblk8 : Constant  Value=[-651680691.972092]  SampleTime=1
  cfblk9 : Constant  Value=[60891814.820936]  SampleTime=1
  cfblk2 : Outport
  cfblk10 : Outport  Port=2
  wires:
  cfblk9/1 -> cfblk3/1
  cfblk8/1 -> cfblk6/1
  cfblk7/1 -> cfblk5/1
  cfblk5/1 -> cfblk10/1
  cfblk3/1 -> cfblk7/1
  cfblk1/1 -> cfblk4/1
  cfblk6/1 -> cfblk2/1

== system sampleModel106/cfblk80/cfblk9/cfblk12/cfblk7 ==
  cfblk1 : Inport
  cfblk10 : Constant  Value=[-457484768.580128]  SampleTime=1
  cfblk11 : Constant  Value=[658100407.685321]  SampleTime=1
  cfblk12 : Constant  Value=[218636306.634220]  SampleTime=1
  cfblk14 : Delay
  cfblk3 : DiscreteFilter
  cfblk4 : UnaryMinus
  cfblk5 : ComplexToRealImag
  cfblk6 : Sum  Inputs=+-
  cfblk7 : MinMax  Function=max
  cfblk8 : Abs  SaturateOnIntegerOverflow=off
  cfblk9 : ComplexToRealImag
  cfblk2 : Outport
  cfblk13 : Outport  Port=2
  wires:
  cfblk9/1 -> cfblk3/1
  cfblk7/1 -> cfblk4/1
  cfblk8/1 -> cfblk13/1
  cfblk1/1 -> cfblk2/1
  cfblk10/1 -> cfblk7/1
  cfblk11/1 -> cfblk8/1
  cfblk5/1 -> cfblk6/1
  cfblk6/1 -> cfblk9/1
  cfblk5/2 -> cfblk6/2
  cfblk9/2 -> cfblk14/1
  cfblk14/1 -> cfblk5/1

== system sampleModel106/cfblk80/cfblk9/cfblk12/cfblk8 ==
  cfblk1 : Inport
  cfblk9 : Inport  Port=2
  cfblk10 : Inport  Port=3
  cfblk11 : Inport  Port=4
  cfblk12 : Inport  Port=5
  cfblk13 : Inport  Port=6
  cfblk3 : simulink/Discrete/Difference  ICPrevInput=0.0  OutMin=[]  OutMax=[]  OutDataTypeStr=Inherit: Inherit via back propagation  OutDataType=fixdt(1, 16)  OutScaling=2^-10  DoSatur=off
  cfblk4 : Product  Inputs=*
  cfblk5 : PermuteDimensions
  cfblk6 : Sum  Inputs=+
  cfblk7 : Abs  SaturateOnIntegerOverflow=off
  cfblk8 : Constant  Value=[734478076.867419]  SampleTime=1
  cfblk2 : Outport
  cfblk14 : Outport  Port=2
  wires:
  cfblk1/1 -> cfblk5/1
  cfblk7/1 -> cfblk3/1
  cfblk8/1 -> cfblk7/1
  cfblk10/1 -> cfblk6/1
  cfblk11/1 -> cfblk2/1
  cfblk12/1 -> cfblk4/1
  cfblk6/1 -> cfblk14/1

== system sampleModel106/cfblk80/cfblk9/cfblk12/cfblk9 ==
  cfblk1 : Inport
  cfblk10 : Signum
  cfblk11 : ComplexToMagnitudeAngle
  cfblk12 : Constant  Value=[-768387414.727406]  SampleTime=1
  cfblk13 : Constant  Value=[275590691.539404]  SampleTime=1
  cfblk14 : Delay
  cfblk3 : Delay  DelayLengthSource=Input port
      settings: InputPortMap=u0,p1
  cfblk4 : slpidlib/PID Controller  Controller=PID  Form=Parallel  TimeDomain=Discrete-time  UseExternalTs=off  SampleTime=-1  IntegratorMethod=Forward Euler  FilterMethod=Forward Euler  ControllerParametersSource=internal  P=1  I=1  UseKiTs=off  D=0  N=100  UseFilter=on  TunerSelectOption=Transfer Function Based (PID Tuner App)  InitialConditionSource=internal  InitialConditionForIntegrator=0  InitialConditionForFilter=0  DifferentiatorICPrevScaledInput=0  ExternalReset=none  TrackingMode=off  Kt=1  LimitOutput=off  SatLimitsSource=internal  UpperSaturationLimit=inf  LowerSaturationLimit=-inf  LinearizeAsGain=off  AntiWindupMode=none  Kb=1  POutMin=[]  POutMax=[]  IOutMin=[]  IOutMax=[]  DOutMin=[]  DOutMax=[]  NOutMin=[]  NOutMax=[]  SumOutMin=[]  SumOutMax=[]  SaturationOutMin=[]  SaturationOutMax=[]  PParamMin=[]  PParamMax=[]  IParamMin=[]  IParamMax=[]  DParamMin=[]  DParamMax=[]  NParamMin=[]  NParamMax=[]  KbParamMin=[]  KbParamMax=[]  KtParamMin=[]  KtParamMax=[]  KbOutMin=[]  KbOutMax=[]  KtOutMin=[]  KtOutMax=[]  IntegratorOutMin=[]  IntegratorOutMax=[]  FilterOutMin=[]  FilterOutMax=[]  SumI1OutMin=[]  SumI1OutMax=[]  SumI2OutMin=[]  SumI2OutMax=[]  SumI3OutMin=[]  SumI3OutMax=[]  SumI4OutMin=[]  SumI4OutMax=[]  SumDOutMin=[]  SumDOutMax=[]  DifferentiatorOutMin=[]  DifferentiatorOutMax=[]  FilterDiffOutCoefMin=[]  FilterDiffOutCoefMax=[]  ReciprocalOutMin=[]  ReciprocalOutMax=[]  SumDenOutMin=[]  SumDenOutMax=[]  SumNumOutMin=[]  SumNumOutMax=[]  DivideOutMin=[]  DivideOutMax=[]  UdiffTsProdOutMin=[]  UdiffTsProdOutMax=[]  NTsProdOutMin=[]  NTsProdOutMax=[]  UintegralTsProdOutMin=[]  UintegralTsProdOutMax=[]  UngainTsProdOutMin=[]  UngainTsProdOutMax=[]  IntegratorContinuousStateAttributes=''  IntegratorStateMustResolveToSignalObject=off  IntegratorRTWStateStorageClass=Auto  FilterContinuousStateAttributes=''  FilterStateMustResolveToSignalObject=off  FilterRTWStateStorageClass=Auto  ParallelPVariant=InternalParameters  IdealPVariant=Disabled  IVariant=InternalParameters  DVariant=InternalParameters  IntegratorVariant=Discrete  SatVariant=Disabled  AWVariant=Passthrough  PCopyVariant=Disabled  TRVariant=Disabled  FdbkBlocksVariant=Forward  IdealPFdbkVariant=Disabled  SatFdbkVariant=Disabled  DerivativeFilterVariant=ForwardEulerFilter  NVariant=InternalParameters  NCopyVariant=Disabled  FilterICVariant=InternalICsFilter  IntegratorICVariant=InternalICs  ExternalResetVariant=Disabled  TRSumVariant=Passthrough  SumFdbkVariant=Disabled  SumVariant=Sum_PID  TsampFilterVariant=InternalTs  TsampNgainVariant=Passthrough  TsampIntegralVariant=Passthrough  ExternalSaturationOutDataTypeStr=Inherit: Same as second input  aMode=0
  cfblk5 : ComplexToMagnitudeAngle
  cfblk6 : simulink/Math Operations/MinMax Running Resettable  Function=min  vinit=0.0
  cfblk7 : UnaryMinus
  cfblk8 : Sin  TimeSource=Use external signal  SampleTime=0
  cfblk9 : Signum
  cfblk2 : Outport
  wires:
  cfblk13/1 -> cfblk6/1
  cfblk12/1 -> cfblk10/1
  cfblk6/1 -> cfblk7/1
  cfblk3/1 -> cfblk2/1
  cfblk10/1 -> cfblk3/1
  cfblk11/1 -> cfblk5/1
  cfblk11/2 -> cfblk8/1
  cfblk8/1 -> cfblk3/2
  cfblk1/1 -> cfblk6/2
  cfblk7/1 -> cfblk11/1
  cfblk4/1 -> cfblk9/1
  cfblk9/1 -> cfblk14/1
  cfblk14/1 -> cfblk4/1

== system sampleModel106/cfblk80/cfblk9/cfblk6/cfblk11 ==
  cfblk1 : Inport
  cfblk12 : Inport  Port=2
  cfblk10 : Constant  Value=[537537931.051630]  SampleTime=1
  cfblk11 : Constant  Value=[-230242735.357014]  SampleTime=1
  cfblk14 : Delay  SampleTime=1
  cfblk3 : UnitDelay  HasFrameUpgradeWarning=on
  cfblk4 : slpidlib/PID Controller  Controller=PID  Form=Parallel  TimeDomain=Discrete-time  UseExternalTs=off  SampleTime=1  IntegratorMethod=Forward Euler  FilterMethod=Forward Euler  ControllerParametersSource=internal  P=1  I=1  UseKiTs=off  D=0  N=100  UseFilter=on  TunerSelectOption=Transfer Function Based (PID Tuner App)  InitialConditionSource=internal  InitialConditionForIntegrator=0  InitialConditionForFilter=0  DifferentiatorICPrevScaledInput=0  ExternalReset=none  TrackingMode=off  Kt=1  LimitOutput=off  SatLimitsSource=internal  UpperSaturationLimit=inf  LowerSaturationLimit=-inf  LinearizeAsGain=off  AntiWindupMode=none  Kb=1  POutMin=[]  POutMax=[]  IOutMin=[]  IOutMax=[]  DOutMin=[]  DOutMax=[]  NOutMin=[]  NOutMax=[]  SumOutMin=[]  SumOutMax=[]  SaturationOutMin=[]  SaturationOutMax=[]  PParamMin=[]  PParamMax=[]  IParamMin=[]  IParamMax=[]  DParamMin=[]  DParamMax=[]  NParamMin=[]  NParamMax=[]  KbParamMin=[]  KbParamMax=[]  KtParamMin=[]  KtParamMax=[]  KbOutMin=[]  KbOutMax=[]  KtOutMin=[]  KtOutMax=[]  IntegratorOutMin=[]  IntegratorOutMax=[]  FilterOutMin=[]  FilterOutMax=[]  SumI1OutMin=[]  SumI1OutMax=[]  SumI2OutMin=[]  SumI2OutMax=[]  SumI3OutMin=[]  SumI3OutMax=[]  SumI4OutMin=[]  SumI4OutMax=[]  SumDOutMin=[]  SumDOutMax=[]  DifferentiatorOutMin=[]  DifferentiatorOutMax=[]  FilterDiffOutCoefMin=[]  FilterDiffOutCoefMax=[]  ReciprocalOutMin=[]  ReciprocalOutMax=[]  SumDenOutMin=[]  SumDenOutMax=[]  SumNumOutMin=[]  SumNumOutMax=[]  DivideOutMin=[]  DivideOutMax=[]  UdiffTsProdOutMin=[]  UdiffTsProdOutMax=[]  NTsProdOutMin=[]  NTsProdOutMax=[]  UintegralTsProdOutMin=[]  UintegralTsProdOutMax=[]  UngainTsProdOutMin=[]  UngainTsProdOutMax=[]  IntegratorContinuousStateAttributes=''  IntegratorStateMustResolveToSignalObject=off  IntegratorRTWStateStorageClass=Auto  FilterContinuousStateAttributes=''  FilterStateMustResolveToSignalObject=off  FilterRTWStateStorageClass=Auto  ParallelPVariant=InternalParameters  IdealPVariant=Disabled  IVariant=InternalParameters  DVariant=InternalParameters  IntegratorVariant=Discrete  SatVariant=Disabled  AWVariant=Passthrough  PCopyVariant=Disabled  TRVariant=Disabled  FdbkBlocksVariant=Forward  IdealPFdbkVariant=Disabled  SatFdbkVariant=Disabled  DerivativeFilterVariant=ForwardEulerFilter  NVariant=InternalParameters  NCopyVariant=Disabled  FilterICVariant=InternalICsFilter  IntegratorICVariant=InternalICs  ExternalResetVariant=Disabled  TRSumVariant=Passthrough  SumFdbkVariant=Disabled  SumVariant=Sum_PID  TsampFilterVariant=InternalTs  TsampNgainVariant=Passthrough  TsampIntegralVariant=Passthrough  ExternalSaturationOutDataTypeStr=Inherit: Same as second input  aMode=0
  cfblk5 : Signum
  cfblk6 : Assignment  DiagnosticForDimensions=Warning  IndexOptions=Index vector (dialog)  Indices=1  OutputSizes=1
  cfblk7 : Rounding
  cfblk8 : Bias  Bias=[-77235819.337838]  SaturateOnIntegerOverflow=off
  cfblk9 : Constant  Value=[-163140347.113187]  SampleTime=1
  cfblk2 : Outport
  cfblk13 : Outport  Port=2
  wires:
  cfblk1/1 -> cfblk4/1
  cfblk5/1 -> cfblk7/1
  cfblk9/1 -> cfblk2/1
  cfblk10/1 -> cfblk8/1
  cfblk12/1 -> cfblk3/1
  cfblk4/1 -> cfblk6/1
  cfblk11/1 -> cfblk13/1
  cfblk3/1 -> cfblk6/2
  cfblk7/1 -> cfblk14/1
  cfblk14/1 -> cfblk5/1

== system sampleModel106/cfblk80/cfblk9/cfblk6/cfblk12 ==
  cfblk1 : Inport
  cfblk11 : Inport  Port=2
  cfblk10 : Constant  Value=[607005750.097917]  SampleTime=1
  cfblk3 : simulink/Discrete/Transfer Fcn Real Zero  ZeroZ=0.75  ICPrevInput=0.0  DoSatur=off
      settings: SourceProductBaseCode=SL
  cfblk4 : DiscreteZeroPole  Poles=[0 0.5]  Gain=1
  cfblk5 : Rounding
  cfblk6 : Rounding
  cfblk7 : Polyval  Coefs=[ +2.081618890e-019, -1.441693666e-014, +4.719686976e-010, -8.536869453e-006, +1.621573104e-001, -8.087801117e+001 ]
  cfblk8 : Trigonometry
  cfblk9 : Sum  Inputs=+
  cfblk2 : Outport
  cfblk12 : Outport  Port=2
  wires:
  cfblk4/1 -> cfblk2/1
  cfblk6/1 -> cfblk9/1
  cfblk8/1 -> cfblk12/1
  cfblk5/1 -> cfblk3/1
  cfblk11/1 -> cfblk6/1
  cfblk7/1 -> cfblk5/1
  cfblk9/1 -> cfblk7/1
  cfblk3/1 -> cfblk4/1
  cfblk10/1 -> cfblk8/1

== system sampleModel106/cfblk80/cfblk9/cfblk6/cfblk13 ==
  cfblk1 : Inport
  cfblk8 : Inport  Port=2
  cfblk9 : Inport  Port=3
  cfblk3 : DiscreteIntegrator  ICPrevOutput=DiscIntNeverNeededParam  ICPrevScaledInput=DiscIntNeverNeededParam
  cfblk4 : Abs  SaturateOnIntegerOverflow=off
  cfblk5 : PermuteDimensions
  cfblk6 : Sqrt
  cfblk7 : Constant  Value=[-963625660.889158]  SampleTime=1
  cfblk2 : Outport
  cfblk10 : Outport  Port=2
  cfblk11 : Outport  Port=3
  wires:
  cfblk9/1 -> cfblk2/1
  cfblk1/1 -> cfblk11/1
  cfblk3/1 -> cfblk10/1
  cfblk8/1 -> cfblk4/1
  cfblk6/1 -> cfblk5/1
  cfblk7/1 -> cfblk3/1
  cfblk4/1 -> cfblk6/1

== system sampleModel106/cfblk80/cfblk9/cfblk6/cfblk14 ==
  cfblk1 : Inport
  cfblk10 : Inport  Port=2
  cfblk11 : Inport  Port=3
  cfblk12 : Inport  Port=4
  cfblk13 : Inport  Port=5
  cfblk14 : Inport  Port=6
  cfblk3 : DiscreteFir  SampleTime=1
  cfblk4 : simulink/Discrete/Difference  ICPrevInput=0.0  OutMin=[]  OutMax=[]  OutDataTypeStr=Inherit: Inherit via back propagation  OutDataType=fixdt(1, 16)  OutScaling=2^-10  DoSatur=off
  cfblk5 : Signum
  cfblk6 : Product  Inputs=*
  cfblk7 : Product
  cfblk8 : Abs  SaturateOnIntegerOverflow=off
  cfblk9 : Constant  Value=[-438303057.716285]  SampleTime=1
  cfblk2 : Outport
  wires:
  cfblk14/1 -> cfblk8/1
  cfblk3/1 -> cfblk4/1
  cfblk5/1 -> cfblk6/1
  cfblk13/1 -> cfblk7/1
  cfblk10/1 -> cfblk5/1
  cfblk4/1 -> cfblk2/1
  cfblk7/1 -> cfblk3/1
  cfblk1/1 -> cfblk7/2
